simulink model "QASKReceiver"  (R2019b)
settings: Solver=VariableStepAuto  StartTime=0.0  StopTime=5  RelTol=1e-3
libraries: commfilt2 x2, dspfdesign x2, commchan3 x1
settings Model: Creator=z3454314  LastModifiedBy=z3454314

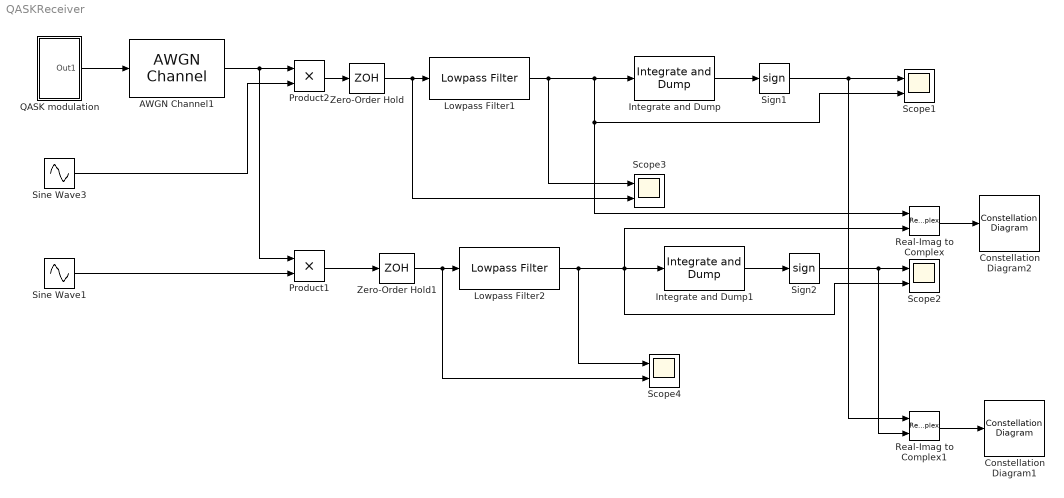
== system QASKReceiver ==
  AWGN Channel1 : commchan3/AWGN Channel  InputProcessing=Columns as channels (frame based)  seed=67  noiseMode="Signal to noise ratio  (SNR)"  EbNodB=30  EsNodB=10  SNRdB=50  bitsPerSym=1  Ps=0.5  Tsym=1/500  variance=1
      settings: SourceProductName=Communications Toolbox
  Constellation Diagram1 : ConstellationDiagram
  Constellation Diagram2 : ConstellationDiagram
  Integrate and Dump : commfilt2/Integrate and Dump  obssamples=250  offsetsamples=23  nodump=off  roundingMode=Floor  overflowMode=off  outputDataTypeStr=Inherit: Same as accumulator  outputLastDataTypeStr=Inherit: Same as accumulator
      settings: SourceProductName=Communications Toolbox
  Integrate and Dump1 : commfilt2/Integrate and Dump  obssamples=250  offsetsamples=23  nodump=off  roundingMode=Floor  overflowMode=off  outputDataTypeStr=Inherit: Same as accumulator  outputLastDataTypeStr=Inherit: Same as accumulator
      settings: SourceProductName=Communications Toolbox
  Lowpass Filter1 : dspfdesign/Lowpass Filter  FilterType=FIR  DesignForMinimumOrder=on  FilterOrder=50  PassbandFrequency=3e3  StopbandFrequency=6e3  PassbandRipple=0.1  StopbandAttenuation=80  InheritSampleRate=on  SampleRate=500e3  SimulateUsing=Interpreted execution  roundingMode=Floor  coeffsDataTypeStr=fixdt(1,16)
  Lowpass Filter2 : dspfdesign/Lowpass Filter  FilterType=FIR  DesignForMinimumOrder=on  FilterOrder=50  PassbandFrequency=3e3  StopbandFrequency=6e3  PassbandRipple=0.1  StopbandAttenuation=80  InheritSampleRate=on  SampleRate=500e3  SimulateUsing=Interpreted execution  roundingMode=Floor  coeffsDataTypeStr=fixdt(1,16)
  Product1 : Product
  Product2 : Product
  QASK modulation : Subsystem
  Real-Imag to Complex : RealImagToComplex
  Real-Imag to Complex1 : RealImagToComplex
  Scope{1..4} (4 alike) : Scope  NumInputPorts=2
  Sign1 : Signum
  Sign2 : Signum
  Sine Wave1 : Sin  Frequency=8000*2*pi  Phase=pi/2  SampleTime=0
  Sine Wave3 : Sin  Frequency=8000*2*pi  SampleTime=0
  Zero-Order Hold : ZeroOrderHold  SampleTime=500e3
  Zero-Order Hold1 : ZeroOrderHold  SampleTime=500e3
  wires:
  QASK modulation/1(Out1) -> AWGN Channel1/1
  AWGN Channel1/1 -> Product1/1, Product2/1
  Sine Wave3/1 -> Product2/2
  Product2/1 -> Zero-Order Hold/1
  Zero-Order Hold/1 -> Scope3/2, Lowpass Filter1/1
  Lowpass Filter1/1 -> Real-Imag to Complex/1, Scope1/2, Integrate and Dump/1, Scope3/1
  Sign1/1 -> Real-Imag to Complex1/1, Scope1/1
  Sine Wave1/1 -> Product1/2
  Product1/1 -> Zero-Order Hold1/1
  Zero-Order Hold1/1 -> Scope4/2, Lowpass Filter2/1
  Sign2/1 -> Real-Imag to Complex1/2, Scope2/1
  Integrate and Dump1/1 -> Sign2/1
  Real-Imag to Complex/1 -> Constellation Diagram2/1
  Lowpass Filter2/1 -> Real-Imag to Complex/2, Scope2/2, Integrate and Dump1/1, Scope4/1
  Real-Imag to Complex1/1 -> Constellation Diagram1/1
  Integrate and Dump/1 -> Sign1/1

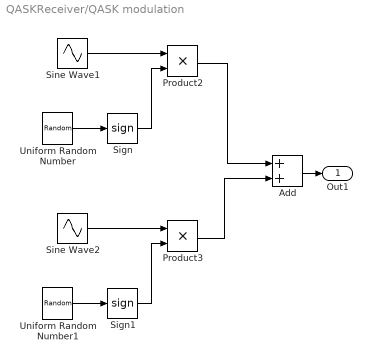
== system QASKReceiver/QASK modulation ==
  Add : Sum
  Product2 : Product
  Product3 : Product
  Sign : Signum
  Sign1 : Signum
  Sine Wave1 : Sin  Frequency=8000*2*pi  SampleTime=0
  Sine Wave2 : Sin  Frequency=8000*2*pi  Phase=pi/2  SampleTime=0
  Uniform Random Number : UniformRandomNumber  SampleTime=1/2000
  Uniform Random Number1 : UniformRandomNumber  Seed=1  SampleTime=1/2000
  Out1 : Outport
  wires:
  Add/1 -> Out1/1
  Uniform Random Number/1 -> Sign/1
  Uniform Random Number1/1 -> Sign1/1
  Product2/1 -> Add/1
  Sign1/1 -> Product3/2
  Sign/1 -> Product2/2
  Product3/1 -> Add/2
  Sine Wave1/1 -> Product2/1
  Sine Wave2/1 -> Product3/1
